simulink model "ev"  (Simulink 8.1)
settings: Solver=ode3  StartTime=0  StopTime=14400  FixedStep=1  RelTol=1e-3
libraries: CampusEnergyModeling x2, powerlib_meascontrol x1
settings Model: Creator=sfrank1  LastModifiedBy=sfrank1
settings DataIOCC: SignalLoggingSaveFormat=Dataset
settings OptimizationCC: ExpressionDepthLimit=128
settings DebuggingCC: FcnCallInpInsideContextMsg=EnableAllAsError
settings GRTTargetCC: CombineOutputUpdateFcns=on  GRTInterface=off

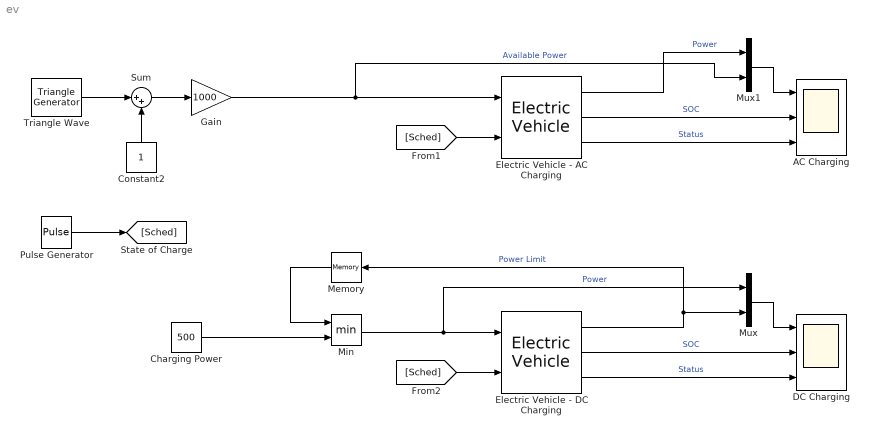
== system ev ==
  AC Charging : Scope  NumInputPorts=3
      settings: ShowLegends=on  TimeRange=15000  YMin=0~0~-1  YMax=2000~1~1
  Charging Power : Constant  Value=500
  Constant2 : Constant
  DC Charging : Scope  NumInputPorts=3
      settings: ShowLegends=on  TimeRange=15000  YMin=0~0~-1  YMax=1000~0.9~0
  Electric Vehicle - AC Charging : CampusEnergyModeling/Electric Vehicles/Electric Vehicle  ctype=AC  rating=1000  chargerEff=0.99  profile=on  profileSOC=[0.00 0.10 0.20 0.80 0.99 1.00]  profileRate=[0.20 0.20 1.00 1.00 0.10 0.10]  capacity=1000  initSOC=0  battEff=0.98
  Electric Vehicle - DC Charging : CampusEnergyModeling/Electric Vehicles/Electric Vehicle  ctype=DC  rating=6240  chargerEff=0.96  profile=off  profileSOC=[0.00 0.10 0.20 0.80 0.99 1.00]  profileRate=[0.10 0.20 1.00 1.00 0.01 0.00]  capacity=1000  initSOC=0  battEff=0.98
  Gain : Gain  Gain=1000
  Memory : Memory
  Min : MinMax  Inputs=2
  Mux : Mux  Inputs=2
  Mux1 : Mux  Inputs=2
  Pulse Generator : DiscretePulseGenerator  PulseType=Time based  Period=9000  PulseWidth=90  PhaseDelay=1800
  Sum : Sum  Inputs=|++
  Triangle Wave : powerlib_meascontrol/Pulse & Signal Generators/Triangle Generator  Freq=1/3600  Phase=0  Ts=0
  wires:
  Electric Vehicle - DC Charging/1 -> Memory/1, Mux/2  "Power Limit"
  Triangle Wave/1 -> Sum/1
  Constant2/1 -> Sum/2
  Sum/1 -> Gain/1
  Gain/1 -> Mux1/2, Electric Vehicle - AC Charging/1  "Available Power"
  Charging Power/1 -> Min/2
  Min/1 -> Mux/1, Electric Vehicle - DC Charging/1  "Power"
  Memory/1 -> Min/1
  Mux/1 -> DC Charging/1
  Electric Vehicle - DC Charging/2 -> DC Charging/2  "SOC"
  Electric Vehicle - DC Charging/3 -> DC Charging/3  "Status"
  Mux1/1 -> AC Charging/1
  Electric Vehicle - AC Charging/2 -> AC Charging/2  "SOC"
  Electric Vehicle - AC Charging/3 -> AC Charging/3  "Status"
  Electric Vehicle - AC Charging/1 -> Mux1/1  "Power"
  [Sched] -> Electric Vehicle - AC Charging/2
  Pulse Generator/1 -> [Sched]
  [Sched] -> Electric Vehicle - DC Charging/2
